simulink model "sim_UAV_Cascada"  (R2015a)
settings: Solver=ode45  StartTime=0.0  StopTime=20  MaxStep=0.001  RelTol=1e-3
values from neighbouring files (symbols this model uses):
  g = 9.81    [Init_UAV.m]    (also in Parametros.m)
  K_pitch = 0.1861    [Parametros.m]
  K_roll = 0.1861    [Parametros.m]
  K_yaw = 2.48    [Parametros.m]
  Kd_pitch = 0.0957    [Parametros.m]
  Kd_roll = 0.0957    [Parametros.m]
  Kd_yaw = 0    [Parametros.m]
  Ki_pitch = 3.69    [Parametros.m]
  Ki_roll = 3.69    [Parametros.m]
  Ki_yaw = 3.77    [Parametros.m]
  KKt = 0.8    [Parametros.m]
  Kphi = 0.4    [Parametros.m]
  Kpsi = 0.3    [Parametros.m]
  Ktheta = 0.4    [Parametros.m]
  l = 0.235    [Init_UAV.m]    (also in Parametros.m)
  m = 0.65    [Init_UAV.m]    (also in Parametros.m = 1.3)
  N = 18    [Parametros.m]
  Nyaw = 10    [Parametros.m]
  tau = 0.06035    [Parametros.m]
  Tt = 1    [Parametros.m]
  Ttyaw = 3.5    [Parametros.m]
undefined symbols (not defined in the file): attitude0, I, omega0, pos0, vel0
libraries: simulink x12, aerolibtransform2 x2, aerolibutil x2
settings Model: Creator=Miguel  LastModifiedBy=Eduardo
settings DataIOCC: SignalLoggingSaveFormat=ModelDataLogs
settings DebuggingCC: SolverPrmCheckMsg=warning  MultiTaskDSMMsg=warning  MultiTaskCondExecSysMsg=none  StrictBusMsg=ErrorOnBusTreatedAsVector

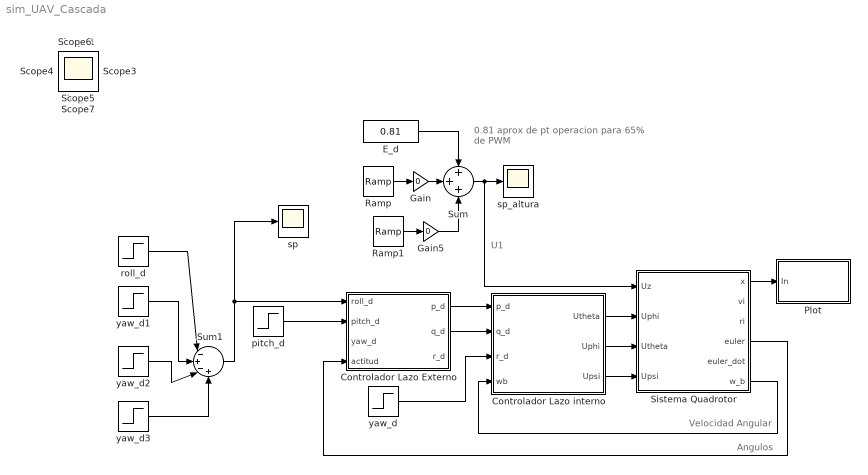
== system sim_UAV_Cascada ==
  note: U1
  note: Angulos
  note: Velocidad Angular
  note: 0.81 aprox
      | de pt operacion para 65% de PWM
  Controlador Lazo Externo : Subsystem
  "Controlador Lazo interno " : Subsystem
  E_d : Constant  Value=0.81
  Gain : Gain  Gain=0
  Gain5 : Gain  Gain=0
  Plot : Subsystem
  Ramp : simulink/Sources/Ramp  slope=1  start=3  X0=0
  Ramp1 : simulink/Sources/Ramp  slope=-1  start=13  X0=0
  Sistema Quadrotor : Subsystem
  Sum : Sum  Inputs=+++
  Sum1 : Sum  Inputs=|-+-+
  pitch_d : Step  Time=0  After=0  SampleTime=0
  roll_d : Step  Time=5  After=25  SampleTime=0
  sp : Scope
      settings: TimeRange=3.666361136571954  YMin=-12.33117816091954  YMax=-8.609913793103445  SaveName=ScopeData21
  sp_altura : Scope
      settings: TimeRange=3.666361136571954  YMin=-12.33117816091954  YMax=-8.609913793103445  SaveName=ScopeData19
  yaw_d : Step  Time=3  After=0  SampleTime=0
  yaw_d1 : Step  Time=7  After=55  SampleTime=0
  yaw_d2 : Step  Time=12  After=50  SampleTime=0
  yaw_d3 : Step  Time=16  After=20  SampleTime=0
  Scope{,1..7} (8 alike) : Scope
      Scope settings: MaxDataPoints=7500
      Scope1 settings: MaxDataPoints=7500
      Scope2 settings: SaveName=ScopeData2  MaxDataPoints=7500
      Scope3 settings: SaveName=ScopeData3  MaxDataPoints=7500
      Scope4 settings: SaveName=ScopeData4  MaxDataPoints=7500
      Scope5 settings: SaveName=ScopeData5  MaxDataPoints=7500
      Scope6 settings: SaveName=ScopeData6  MaxDataPoints=7500
      Scope7 settings: SaveName=ScopeData7  MaxDataPoints=7500
  wires:
  Sistema Quadrotor/1(x) -> Plot/1(In)
  Controlador Lazo Externo/1(p_d) -> "Controlador Lazo interno "/1(p_d)
  Controlador Lazo Externo/2(q_d) -> "Controlador Lazo interno "/2(q_d)
  pitch_d/1 -> Controlador Lazo Externo/2(pitch_d)
  yaw_d1/1 -> Sum1/2
  yaw_d2/1 -> Sum1/3
  yaw_d3/1 -> Sum1/4
  Sistema Quadrotor/6(w_b) -> "Controlador Lazo interno "/4(wb)
  Sistema Quadrotor/4(euler) -> Controlador Lazo Externo/4(actitud)
  E_d/1 -> Sum/1
  Sum/1 -> Sistema Quadrotor/1(Uz), sp_altura/1
  Gain/1 -> Sum/2
  Ramp/1 -> Gain/1
  Ramp1/1 -> Gain5/1
  Gain5/1 -> Sum/3
  "Controlador Lazo interno "/1(Utheta) -> Sistema Quadrotor/2(Uphi)
  "Controlador Lazo interno "/2(Uphi) -> Sistema Quadrotor/3("Utheta ")
  "Controlador Lazo interno "/3(Upsi) -> Sistema Quadrotor/4(Upsi)
  Sum1/1 -> Controlador Lazo Externo/1(roll_d), sp/1
  yaw_d/1 -> "Controlador Lazo interno "/3(r_d)
  roll_d/1 -> Sum1/1

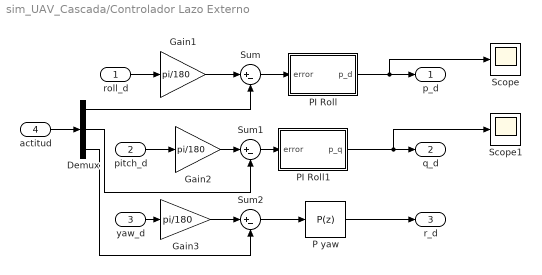
== system sim_UAV_Cascada/Controlador Lazo Externo ==
  roll_d : Inport
  pitch_d : Inport  Port=2
  yaw_d : Inport  Port=3
  actitud : Inport  Port=4
  Demux : Demux  Outputs=3
  Gain1 : Gain  Gain=pi/180
  Gain2 : Gain  Gain=pi/180
  Gain3 : Gain  Gain=pi/180
  P yaw : simulink/Continuous/PID Controller  Controller=P  TimeDomain=Discrete-time  SampleTime=0.01  IntegratorMethod=Forward Euler  FilterMethod=Forward Euler  Form=Parallel  UseFilter=on  ControllerParametersSource=internal  P=4  I=1.5  D=0.00989768140502374  N=2166.61961334261  InitialConditionSource=internal  InitialConditionForIntegrator=0  InitialConditionForFilter=0  ExternalReset=none  LimitOutput=off  UpperSaturationLimit=1.555  LowerSaturationLimit=-1.552  LinearizeAsGain=on  AntiWindupMode=back-calculation  Kb=1  TrackingMode=off  Kt=1  PParamMin=[]  PParamMax=[]  IParamMin=[]  IParamMax=[]  DParamMin=[]  DParamMax=[]  NParamMin=[]  NParamMax=[]  KbParamMin=[]  KbParamMax=[]  KtParamMin=[]  KtParamMax=[]  POutMin=[]  POutMax=[]  IOutMin=[]  IOutMax=[]  DOutMin=[]  DOutMax=[]  NOutMin=[]  NOutMax=[]  KbOutMin=[]  KbOutMax=[]  KtOutMin=[]  KtOutMax=[]  IntegratorOutMin=[]  IntegratorOutMax=[]  FilterOutMin=[]  FilterOutMax=[]  SumOutMin=[]  SumOutMax=[]  SumI1OutMin=[]  SumI1OutMax=[]  SumI2OutMin=[]  SumI2OutMax=[]  SumI3OutMin=[]  SumI3OutMax=[]  SumDOutMin=[]  SumDOutMax=[]  SaturationOutMin=[]  SaturationOutMax=[]  IntegratorContinuousStateAttributes=''  IntegratorStateMustResolveToSignalObject=off  IntegratorRTWStateStorageClass=Auto  FilterContinuousStateAttributes=''  FilterStateMustResolveToSignalObject=off  FilterRTWStateStorageClass=Auto  DifferentiatorICPrevScaledInput=0  DifferentiatorOutMin=[]  DifferentiatorOutMax=[]
  PI Roll : Subsystem
  PI Roll1 : Subsystem
  Scope : Scope
      settings: SaveName=ScopeData27
  Scope1 : Scope
      settings: SaveName=ScopeData28
  Sum : Sum  Inputs=|+-
  Sum1 : Sum  Inputs=|+-
  Sum2 : Sum  Inputs=|+-
  p_d : Outport
  q_d : Outport  Port=2
  r_d : Outport  Port=3
  wires:
  PI Roll1/1(p_q) -> Scope1/1, q_d/1
  P yaw/1 -> r_d/1
  actitud/1 -> Demux/1
  roll_d/1 -> Gain1/1
  pitch_d/1 -> Gain2/1
  yaw_d/1 -> Gain3/1
  Demux/1 -> Sum/2
  Demux/2 -> Sum1/2
  Demux/3 -> Sum2/2
  Sum2/1 -> P yaw/1
  Gain1/1 -> Sum/1
  Gain2/1 -> Sum1/1
  Gain3/1 -> Sum2/1
  Sum/1 -> PI Roll/1(error)
  PI Roll/1(p_d) -> Scope/1, p_d/1
  Sum1/1 -> PI Roll1/1(error)

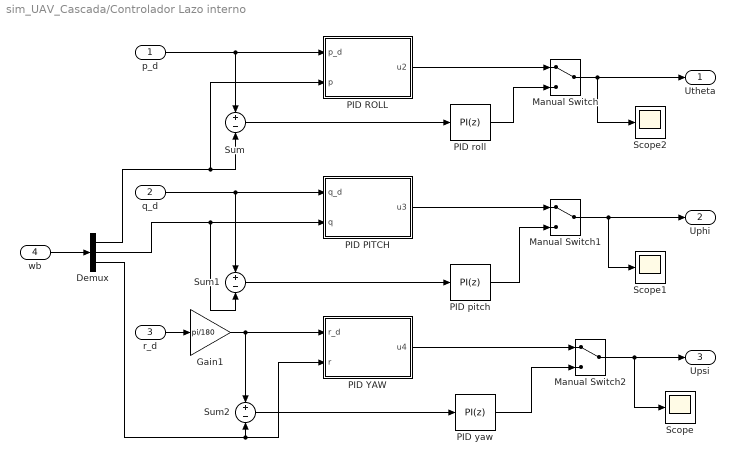
== system sim_UAV_Cascada/Controlador Lazo interno  ==
  p_d : Inport
  q_d : Inport  Port=2
  r_d : Inport  Port=3
  wb : Inport  Port=4
  Demux : Demux  Outputs=3
  Gain1 : Gain  Gain=pi/180
  Manual Switch : ManualSwitch
  Manual Switch1 : ManualSwitch
  Manual Switch2 : ManualSwitch
  PID PITCH : Subsystem
  PID ROLL : Subsystem
  PID YAW : Subsystem
  PID pitch : simulink/Continuous/PID Controller  Controller=PI  TimeDomain=Discrete-time  SampleTime=0.01  IntegratorMethod=Forward Euler  FilterMethod=Forward Euler  Form=Ideal  UseFilter=on  ControllerParametersSource=internal  P=0.09  I=1/0.85  D=0.08  N=10  InitialConditionSource=internal  InitialConditionForIntegrator=0  InitialConditionForFilter=0  ExternalReset=none  LimitOutput=on  UpperSaturationLimit=1  LowerSaturationLimit=-1  LinearizeAsGain=on  AntiWindupMode=back-calculation  Kb=1  TrackingMode=off  Kt=1  PParamMin=[]  PParamMax=[]  IParamMin=[]  IParamMax=[]  DParamMin=[]  DParamMax=[]  NParamMin=[]  NParamMax=[]  KbParamMin=[]  KbParamMax=[]  KtParamMin=[]  KtParamMax=[]  POutMin=[]  POutMax=[]  IOutMin=[]  IOutMax=[]  DOutMin=[]  DOutMax=[]  NOutMin=[]  NOutMax=[]  KbOutMin=[]  KbOutMax=[]  KtOutMin=[]  KtOutMax=[]  IntegratorOutMin=[]  IntegratorOutMax=[]  FilterOutMin=[]  FilterOutMax=[]  SumOutMin=[]  SumOutMax=[]  SumI1OutMin=[]  SumI1OutMax=[]  SumI2OutMin=[]  SumI2OutMax=[]  SumI3OutMin=[]  SumI3OutMax=[]  SumDOutMin=[]  SumDOutMax=[]  SaturationOutMin=[]  SaturationOutMax=[]  IntegratorContinuousStateAttributes=''  IntegratorStateMustResolveToSignalObject=off  IntegratorRTWStateStorageClass=Auto  FilterContinuousStateAttributes=''  FilterStateMustResolveToSignalObject=off  FilterRTWStateStorageClass=Auto  DifferentiatorICPrevScaledInput=0  DifferentiatorOutMin=[]  DifferentiatorOutMax=[]
  PID roll : simulink/Continuous/PID Controller  Controller=PI  TimeDomain=Discrete-time  SampleTime=0.01  IntegratorMethod=Forward Euler  FilterMethod=Forward Euler  Form=Ideal  UseFilter=on  ControllerParametersSource=internal  P=0.09  I=1/0.85  D=0.025  N=10  InitialConditionSource=internal  InitialConditionForIntegrator=0  InitialConditionForFilter=0  ExternalReset=none  LimitOutput=on  UpperSaturationLimit=1  LowerSaturationLimit=-1  LinearizeAsGain=on  AntiWindupMode=back-calculation  Kb=1  TrackingMode=off  Kt=1  PParamMin=[]  PParamMax=[]  IParamMin=[]  IParamMax=[]  DParamMin=[]  DParamMax=[]  NParamMin=[]  NParamMax=[]  KbParamMin=[]  KbParamMax=[]  KtParamMin=[]  KtParamMax=[]  POutMin=[]  POutMax=[]  IOutMin=[]  IOutMax=[]  DOutMin=[]  DOutMax=[]  NOutMin=[]  NOutMax=[]  KbOutMin=[]  KbOutMax=[]  KtOutMin=[]  KtOutMax=[]  IntegratorOutMin=[]  IntegratorOutMax=[]  FilterOutMin=[]  FilterOutMax=[]  SumOutMin=[]  SumOutMax=[]  SumI1OutMin=[]  SumI1OutMax=[]  SumI2OutMin=[]  SumI2OutMax=[]  SumI3OutMin=[]  SumI3OutMax=[]  SumDOutMin=[]  SumDOutMax=[]  SaturationOutMin=[]  SaturationOutMax=[]  IntegratorContinuousStateAttributes=''  IntegratorStateMustResolveToSignalObject=off  IntegratorRTWStateStorageClass=Auto  FilterContinuousStateAttributes=''  FilterStateMustResolveToSignalObject=off  FilterRTWStateStorageClass=Auto  DifferentiatorICPrevScaledInput=0  DifferentiatorOutMin=[]  DifferentiatorOutMax=[]
  PID yaw : simulink/Continuous/PID Controller  Controller=PI  TimeDomain=Discrete-time  SampleTime=0.01  IntegratorMethod=Forward Euler  FilterMethod=Forward Euler  Form=Ideal  UseFilter=on  ControllerParametersSource=internal  P=2.48  I=0.26  D=0.09571  N=189.5  InitialConditionSource=internal  InitialConditionForIntegrator=0  InitialConditionForFilter=0  ExternalReset=none  LimitOutput=on  UpperSaturationLimit=1  LowerSaturationLimit=-1  LinearizeAsGain=on  AntiWindupMode=back-calculation  Kb=3.5  TrackingMode=off  Kt=1  PParamMin=[]  PParamMax=[]  IParamMin=[]  IParamMax=[]  DParamMin=[]  DParamMax=[]  NParamMin=[]  NParamMax=[]  KbParamMin=[]  KbParamMax=[]  KtParamMin=[]  KtParamMax=[]  POutMin=[]  POutMax=[]  IOutMin=[]  IOutMax=[]  DOutMin=[]  DOutMax=[]  NOutMin=[]  NOutMax=[]  KbOutMin=[]  KbOutMax=[]  KtOutMin=[]  KtOutMax=[]  IntegratorOutMin=[]  IntegratorOutMax=[]  FilterOutMin=[]  FilterOutMax=[]  SumOutMin=[]  SumOutMax=[]  SumI1OutMin=[]  SumI1OutMax=[]  SumI2OutMin=[]  SumI2OutMax=[]  SumI3OutMin=[]  SumI3OutMax=[]  SumDOutMin=[]  SumDOutMax=[]  SaturationOutMin=[]  SaturationOutMax=[]  IntegratorContinuousStateAttributes=''  IntegratorStateMustResolveToSignalObject=off  IntegratorRTWStateStorageClass=Auto  FilterContinuousStateAttributes=''  FilterStateMustResolveToSignalObject=off  FilterRTWStateStorageClass=Auto  DifferentiatorICPrevScaledInput=0  DifferentiatorOutMin=[]  DifferentiatorOutMax=[]
  Scope : Scope
      settings: YMin=0.13  YMax=0.36  SaveName=ScopeData13
  Scope1 : Scope
      settings: SaveName=ScopeData14
  Scope2 : Scope
      settings: TimeRange=16  YMin=0  YMax=0.00014  SaveName=ScopeData15
  Sum : Sum  Inputs=+-
  Sum1 : Sum  Inputs=+-
  Sum2 : Sum  Inputs=+-
  Utheta : Outport
  Uphi : Outport  Port=2
  Upsi : Outport  Port=3
  wires:
  Manual Switch2/1 -> Upsi/1, Scope/1
  Manual Switch/1 -> Utheta/1, Scope2/1
  Manual Switch1/1 -> Uphi/1, Scope1/1
  wb/1 -> Demux/1
  p_d/1 -> PID ROLL/1(p_d), Sum/1
  q_d/1 -> Sum1/1, PID PITCH/1(q_d)
  Demux/1 -> PID ROLL/2(p), Sum/2
  Demux/2 -> Sum1/2, PID PITCH/2(q)
  Demux/3 -> PID YAW/2(r), Sum2/2
  Sum/1 -> PID roll/1
  PID pitch/1 -> Manual Switch1/2
  Sum1/1 -> PID pitch/1
  Sum2/1 -> PID yaw/1
  PID yaw/1 -> Manual Switch2/2
  PID roll/1 -> Manual Switch/2
  PID PITCH/1(u3) -> Manual Switch1/1
  PID ROLL/1(u2) -> Manual Switch/1
  PID YAW/1(u4) -> Manual Switch2/1
  r_d/1 -> Gain1/1
  Gain1/1 -> Sum2/1, PID YAW/1(r_d)

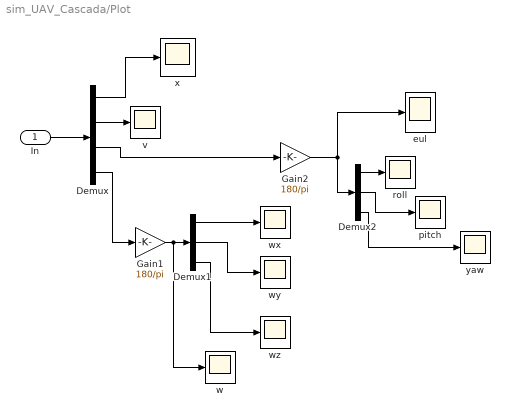
== system sim_UAV_Cascada/Plot ==
  In : Inport
  Demux : Demux
  Demux1 : Demux  Outputs=3
  Demux2 : Demux  Outputs=3
  Gain1 : Gain  Gain=180/pi
  Gain2 : Gain  Gain=180/pi
  eul : Scope
      settings: TimeRange=8  SaveName=ScopeData2
  pitch : Scope
      settings: TimeRange=10  YMin=-0.01  YMax=0.09000000000000001  SaveName=ScopeData12
  roll : Scope
      settings: SaveName=ScopeData10
  v : Scope
  w : Scope
      settings: SaveName=ScopeData25
  wx : Scope
      settings: SaveName=ScopeData3
  wy : Scope
      settings: SaveName=ScopeData23
  wz : Scope
      settings: SaveName=ScopeData24
  x : Scope
  yaw : Scope
      settings: SaveName=ScopeData11
  wires:
  In/1 -> Demux/1
  Demux/1 -> x/1
  Demux/2 -> v/1
  Demux/3 -> Gain2/1
  Gain2/1 -> eul/1, Demux2/1
  Demux2/1 -> roll/1
  Demux2/2 -> pitch/1
  Demux2/3 -> yaw/1
  Demux/4 -> Gain1/1
  Demux1/1 -> wx/1
  Gain1/1 -> w/1, Demux1/1
  Demux1/2 -> wy/1
  Demux1/3 -> wz/1

== system sim_UAV_Cascada/Sistema Quadrotor ==
  Uz : Inport
  Uphi : Inport  Port=2
  "Utheta " : Inport  Port=3
  Upsi : Inport  Port=4
  ACTUADORES : Subsystem
  AERODINÁMICAS : Subsystem
  DINÁMICA QUADROTOR : Subsystem
      mask Display:
      | image(imread('F450.jpg'))
      | port_label('input',1,'{F}^{b} (N)','texmode','on')
      | port_label('input',2,'{M}^{b} (N-m)','texmode','on')
      | port_label('output',1,'x ','texmode','on')
      | port_label('output',2,'{v}^{i} (m/s)','texmode','on')
      | port_label('output',3,'{r}^{i} (m)','texmode','on')
      | port_label('output',4,'\phi \theta \psi (rad)','texmode','on')
      | port_label('output',5,'d[\phi \theta \psi]/dt (rad)','texmode','on')
  MATRIZ DE CONVERSION PWM : Subsystem
  x : Outport
  vi : Outport  Port=2
  ri : Outport  Port=3
  euler : Outport  Port=4
  euler_dot : Outport  Port=5
  w_b : Outport  Port=6
  wires:
  DINÁMICA QUADROTOR/2(v) -> vi/1
  DINÁMICA QUADROTOR/1(estados) -> x/1
  DINÁMICA QUADROTOR/4(eul) -> euler/1
  ACTUADORES/1(Ti) -> AERODINÁMICAS/1(Ti)
  AERODINÁMICAS/1(Fb) -> DINÁMICA QUADROTOR/1(Fuerza)
  AERODINÁMICAS/2(Mb) -> DINÁMICA QUADROTOR/2(Momento)
  DINÁMICA QUADROTOR/3(pos) -> ri/1
  DINÁMICA QUADROTOR/5(Deul) -> euler_dot/1
  DINÁMICA QUADROTOR/6(w_b) -> w_b/1
  ACTUADORES/2(Mi) -> AERODINÁMICAS/2(Mi)
  Uphi/1 -> MATRIZ DE CONVERSION PWM/2(Uphi)
  Uz/1 -> MATRIZ DE CONVERSION PWM/1(Uz)
  "Utheta "/1 -> MATRIZ DE CONVERSION PWM/3(Utheta)
  Upsi/1 -> MATRIZ DE CONVERSION PWM/4(Upsi)
  MATRIZ DE CONVERSION PWM/1(PWM%) -> ACTUADORES/1(PWM%)

== system sim_UAV_Cascada/Controlador Lazo Externo/PI Roll ==
  note: error
  error : Inport
  Integrator : Integrator
  K : Gain  Gain=6
  Sum6 : Sum  Inputs=|++
  Ti : Gain  Gain=0.5
  p_d : Outport
  wires:
  error/1 -> Ti/1, K/1
  K/1 -> Sum6/1
  Ti/1 -> Integrator/1
  Integrator/1 -> Sum6/2
  Sum6/1 -> p_d/1

== system sim_UAV_Cascada/Controlador Lazo Externo/PI Roll1 ==
  note: error
  error : Inport
  Integrator : Integrator
  K : Gain  Gain=6
  Sum6 : Sum  Inputs=|++
  Ti : Gain  Gain=0.5
  p_q : Outport
  wires:
  error/1 -> Ti/1, K/1
  K/1 -> Sum6/1
  Ti/1 -> Integrator/1
  Integrator/1 -> Sum6/2
  Sum6/1 -> p_q/1

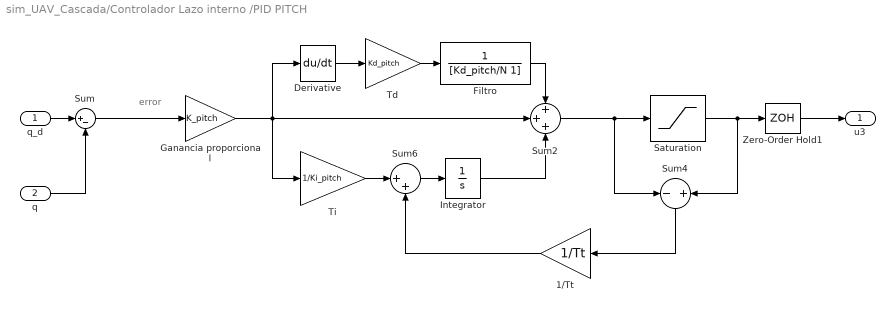
== system sim_UAV_Cascada/Controlador Lazo interno /PID PITCH ==
  note: error
  q_d : Inport
  q : Inport  Port=2
  1/Tt : Gain  Gain=1/Tt
  Derivative : Derivative
  Filtro : TransferFcn  Denominator=[Kd_pitch/N 1]
  Ganancia proporcional : Gain  Gain=K_pitch
  Integrator : Integrator
  Saturation : Saturate  UpperLimit=1  LowerLimit=-1
  Sum : Sum  Inputs=|+-
  Sum2 : Sum  Inputs=+++
  Sum4 : Sum  Inputs=-|+
  Sum6 : Sum  Inputs=|++
  Td : Gain  Gain=Kd_pitch
  Ti : Gain  Gain=1/Ki_pitch
  Zero-Order Hold1 : ZeroOrderHold  SampleTime=0.01
  u3 : Outport
  wires:
  q/1 -> Sum/2
  Sum6/1 -> Integrator/1
  Ganancia proporcional/1 -> Sum2/2, Derivative/1, Ti/1
  Derivative/1 -> Td/1
  Sum4/1 -> 1/Tt/1
  Saturation/1 -> Sum4/2, Zero-Order Hold1/1
  Sum2/1 -> Sum4/1, Saturation/1
  q_d/1 -> Sum/1
  Sum/1 -> Ganancia proporcional/1
  Ti/1 -> Sum6/1
  1/Tt/1 -> Sum6/2
  Td/1 -> Filtro/1
  Integrator/1 -> Sum2/3
  Filtro/1 -> Sum2/1
  Zero-Order Hold1/1 -> u3/1

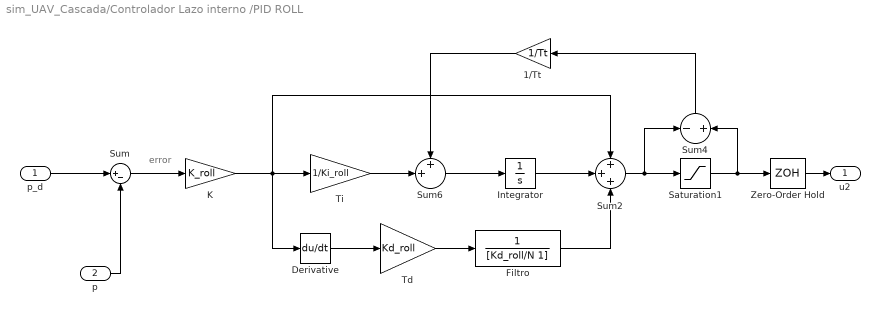
== system sim_UAV_Cascada/Controlador Lazo interno /PID ROLL ==
  note: error
  p_d : Inport
  p : Inport  Port=2
  1/Tt : Gain  Gain=1/Tt
  Derivative : Derivative
  Filtro : TransferFcn  Denominator=[Kd_roll/N 1]
  Integrator : Integrator
  K : Gain  Gain=K_roll
  Saturation1 : Saturate  UpperLimit=1  LowerLimit=-1
  Sum : Sum  Inputs=|+-
  Sum2 : Sum  Inputs=+++
  Sum4 : Sum  Inputs=-+
  Sum6 : Sum  Inputs=++|
  Td : Gain  Gain=Kd_roll
  Ti : Gain  Gain=1/Ki_roll
  Zero-Order Hold : ZeroOrderHold  SampleTime=0.01
  u2 : Outport
  wires:
  p/1 -> Sum/2
  1/Tt/1 -> Sum6/1
  Sum6/1 -> Integrator/1
  K/1 -> Derivative/1, Ti/1, Sum2/1
  Derivative/1 -> Td/1
  Filtro/1 -> Sum2/3
  Td/1 -> Filtro/1
  Integrator/1 -> Sum2/2
  Ti/1 -> Sum6/2
  Sum4/1 -> 1/Tt/1
  Sum2/1 -> Sum4/1, Saturation1/1
  p_d/1 -> Sum/1
  Sum/1 -> K/1
  Saturation1/1 -> Sum4/2, Zero-Order Hold/1
  Zero-Order Hold/1 -> u2/1

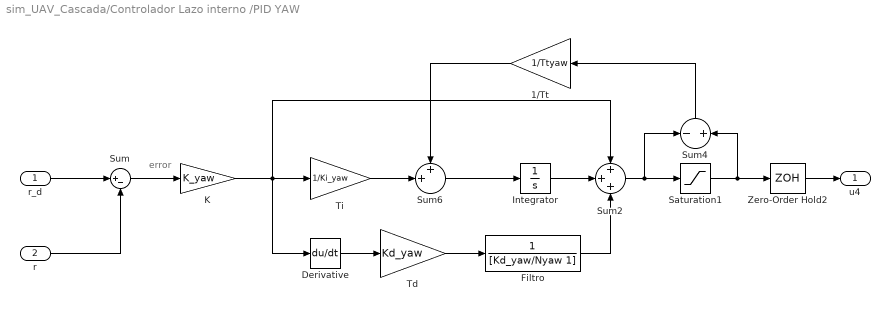
== system sim_UAV_Cascada/Controlador Lazo interno /PID YAW ==
  note: error
  r_d : Inport
  r : Inport  Port=2
  1/Tt : Gain  Gain=1/Ttyaw
  Derivative : Derivative
  Filtro : TransferFcn  Denominator=[Kd_yaw/Nyaw 1]
  Integrator : Integrator
  K : Gain  Gain=K_yaw
  Saturation1 : Saturate  UpperLimit=1  LowerLimit=-1
  Sum : Sum  Inputs=|+-
  Sum2 : Sum  Inputs=+++
  Sum4 : Sum  Inputs=-+
  Sum6 : Sum  Inputs=++|
  Td : Gain  Gain=Kd_yaw
  Ti : Gain  Gain=1/Ki_yaw
  Zero-Order Hold2 : ZeroOrderHold  SampleTime=0.01
  u4 : Outport
  wires:
  r/1 -> Sum/2
  1/Tt/1 -> Sum6/1
  Sum6/1 -> Integrator/1
  K/1 -> Derivative/1, Ti/1, Sum2/1
  Derivative/1 -> Td/1
  Filtro/1 -> Sum2/3
  Td/1 -> Filtro/1
  Integrator/1 -> Sum2/2
  Ti/1 -> Sum6/2
  Sum4/1 -> 1/Tt/1
  Saturation1/1 -> Zero-Order Hold2/1, Sum4/2
  Sum2/1 -> Sum4/1, Saturation1/1
  r_d/1 -> Sum/1
  Sum/1 -> K/1
  Zero-Order Hold2/1 -> u4/1

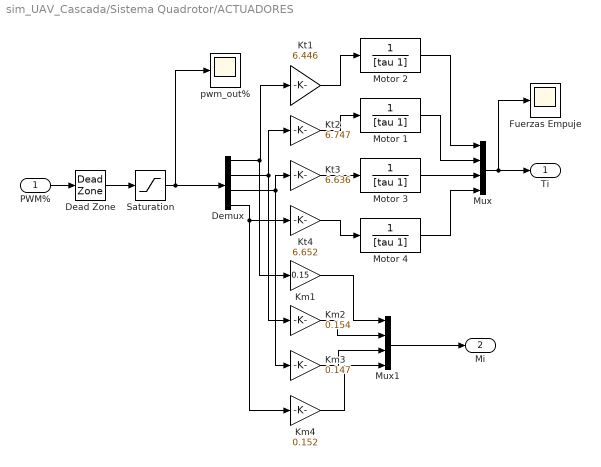
== system sim_UAV_Cascada/Sistema Quadrotor/ACTUADORES ==
  PWM% : Inport
  Dead Zone : DeadZone  LowerValue=0  UpperValue=0.13  SaturateOnIntegerOverflow=on
  Demux : Demux
  Fuerzas Empuje : Scope
      settings: SaveName=ScopeData20
  Km1 : Gain  Gain=0.15
  Km2 : Gain  Gain=0.154
  Km3 : Gain  Gain=0.147
  Km4 : Gain  Gain=0.152
  Kt1 : Gain  Gain=6.446
  Kt2 : Gain  Gain=6.747
  Kt3 : Gain  Gain=6.636
  Kt4 : Gain  Gain=6.652
  Motor {1..4} (4 alike) : TransferFcn  Denominator=[tau 1]
  Mux : Mux
  Mux1 : Mux
  Saturation : Saturate  UpperLimit=1  LowerLimit=0  ZeroCross=off
  pwm_out% : Scope
      settings: SaveName=ScopeData22
  Ti : Outport
  Mi : Outport  Port=2
  wires:
  PWM%/1 -> Dead Zone/1
  Dead Zone/1 -> Saturation/1
  Saturation/1 -> Demux/1, pwm_out%/1
  Demux/1 -> Km1/1, Kt1/1
  Demux/2 -> Km2/1, Kt2/1
  Demux/3 -> Kt3/1, Km3/1
  Demux/4 -> Km4/1, Kt4/1
  Km1/1 -> Mux1/1
  Km2/1 -> Mux1/2
  Km3/1 -> Mux1/3
  Km4/1 -> Mux1/4
  Mux1/1 -> Mi/1
  Kt4/1 -> Motor 4/1
  Kt3/1 -> Motor 3/1
  Kt2/1 -> Motor 1/1
  Kt1/1 -> Motor 2/1
  Motor 2/1 -> Mux/1
  Motor 1/1 -> Mux/2
  Motor 3/1 -> Mux/3
  Motor 4/1 -> Mux/4
  Mux/1 -> Fuerzas Empuje/1, Ti/1

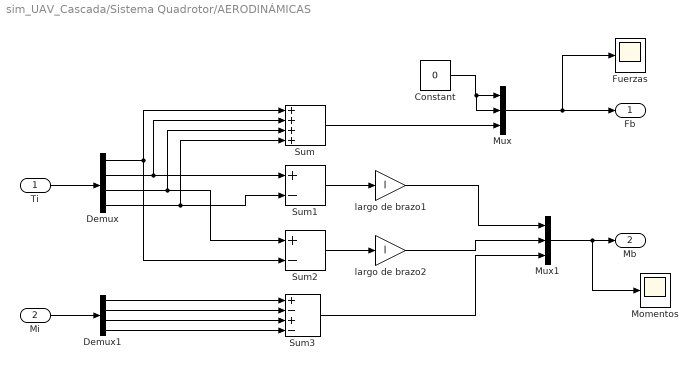
== system sim_UAV_Cascada/Sistema Quadrotor/AERODINÁMICAS ==
  Ti : Inport
  Mi : Inport  Port=2
  Constant : Constant  Value=0
  Demux : Demux
  Demux1 : Demux
  Fuerzas : Scope
      settings: SaveName=ScopeData4
  Momentos : Scope
      settings: SaveName=ScopeData8
  Mux : Mux  Inputs=3
  Mux1 : Mux  Inputs=3
  Sum : Sum  Inputs=++++
  Sum1 : Sum  Inputs=+-
  Sum2 : Sum  Inputs=+-
  Sum3 : Sum  Inputs=+-+-
  largo de brazo1 : Gain  Gain=l
  largo de brazo2 : Gain  Gain=l
  Fb : Outport
  Mb : Outport  Port=2
  wires:
  Ti/1 -> Demux/1
  Mi/1 -> Demux1/1
  Demux/1 -> Sum2/2, Sum/1
  Demux/2 -> Sum1/1, Sum/2
  Demux/3 -> Sum2/1, Sum/3
  Demux/4 -> Sum1/2, Sum/4
  Demux1/1 -> Sum3/1
  Demux1/2 -> Sum3/2
  Demux1/3 -> Sum3/3
  Demux1/4 -> Sum3/4
  Sum1/1 -> largo de brazo1/1
  Sum2/1 -> largo de brazo2/1
  Constant/1 -> Mux/2, Mux/1
  Mux/1 -> Fb/1, Fuerzas/1
  Sum/1 -> Mux/3
  largo de brazo1/1 -> Mux1/1
  largo de brazo2/1 -> Mux1/2
  Sum3/1 -> Mux1/3
  Mux1/1 -> Momentos/1, Mb/1

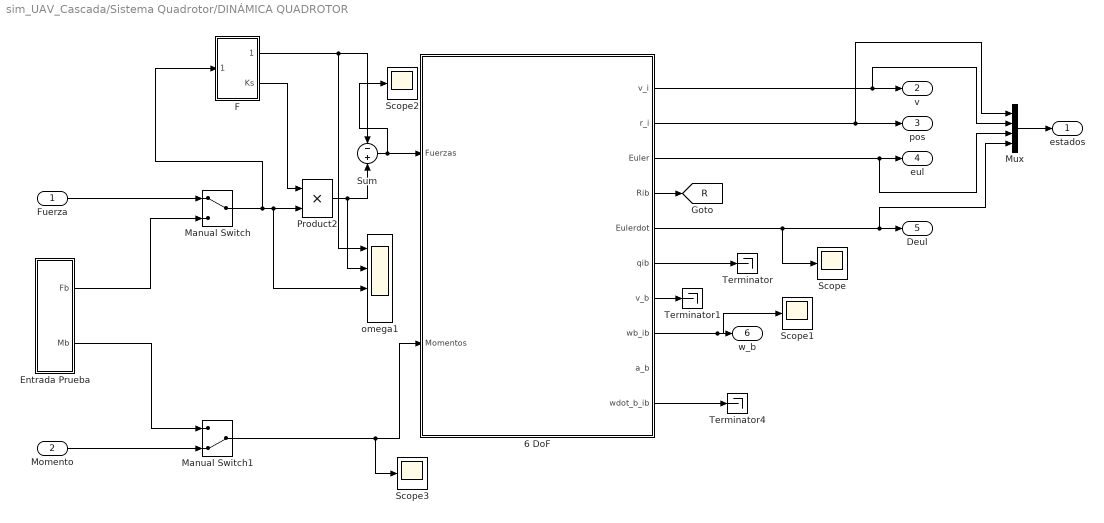
== system sim_UAV_Cascada/Sistema Quadrotor/DINÁMICA QUADROTOR ==
  Fuerza : Inport
  Momento : Inport  Port=2
  6 DoF : Subsystem  mask(Sistema Cuadrirotor){masa=m, Inercia=I, v0_b=vel0, w0b_ib=omega0, r0_i=pos0, eul_0=attitude0}
      mask prompts: masa "masa (Kg) :"; Inercia "Inercia :"; v0_b "Velocidad lineal inicial en el body (m/s):"; w0b_ib "Velocidad angular inicial en el body (rad/s) :"; r0_i "Posición inicial en el inercial (m) :"; eul_0 "Angulos de euler iniciales"
      mask help: Modelo cinemático y dinámico de un UAV tipo Cuadrirotor
      mask Display:
      | port_label('input',1,'{F}^{b} (N)','texmode','on')
      | port_label('input',2,'{M}^{b} (N-m)','texmode','on')
      | port_label('output',1,'{v}^{i} (m/s)','texmode','on')
      | port_label('output',2,'{r}^{i} (m)','texmode','on')
      | port_label('output',3,'\phi \theta \psi (rad)','texmode','on')
      | port_label('output',4,'{R}^{i}_{b}','texmode','on')
      | port_label('output',5,'d[\phi \theta \psi]/dt (rad)','texmode','on')
      | port_label('output',6,'{q}^{i}_{b}','texmode','on')
      | port_label('output',7,'{v}^{b} (m/s)','texmode','on')
      | port_label('output',8,'{\omega}^{b}_{bi} (rad)','texmode','on')
      | port_label('output',9,'{a}^{b} (m/{s}^{2})','texmode','on')
      | port_label('output',10,'d({\omega}^{b}_{ib})/dt (rad/{s}^{2})','texmode','on')
  Entrada Prueba : Subsystem
  F : Subsystem
  Manual Switch : ManualSwitch
  Manual Switch1 : ManualSwitch  CurrentSetting=0
  Mux : Mux
  Product2 : Product
  Scope{,1..3} (4 alike) : Scope
      Scope settings: SaveName=ScopeData16
      Scope1 settings: SaveName=ScopeData17
      Scope2 settings: SaveName=ScopeData18
      Scope3 settings: SaveName=ScopeData26
  Sum : Sum  Inputs=-|+
  Terminator : Terminator
  Terminator1 : Terminator
  Terminator4 : Terminator
  omega1 : Scope  NumInputPorts=4
      settings: YMin=-1~-20~-20~-5  YMax=12~0~0~5  SaveName=ScopeData9
  estados : Outport
  v : Outport  Port=2
  pos : Outport  Port=3
  eul : Outport  Port=4
  Deul : Outport  Port=5
  w_b : Outport  Port=6
  tag scope: R=global
  wires:
  6 DoF/2(r_i) -> pos/1, Mux/1
  6 DoF/4(Rib) -> [R]
  6 DoF/6(qib) -> Terminator/1
  6 DoF/5(Eulerdot) -> Mux/4, Deul/1, Scope/1
  6 DoF/3(Euler) -> Mux/3, eul/1
  Sum/1 -> Scope2/1, 6 DoF/1(Fuerzas)
  6 DoF/10(wdot_b_ib) -> Terminator4/1
  6 DoF/1(v_i) -> Mux/2, v/1
  6 DoF/7(v_b) -> Terminator1/1
  6 DoF/8(wb_ib) -> Scope1/1, w_b/1
  Mux/1 -> estados/1
  Entrada Prueba/1(Fb) -> Manual Switch/2
  Entrada Prueba/2(Mb) -> Manual Switch1/1
  Fuerza/1 -> Manual Switch/1
  Momento/1 -> Manual Switch1/2
  Manual Switch1/1 -> Scope3/1, 6 DoF/2(Momentos)
  Manual Switch/1 -> omega1/3, Product2/2, F/1(Fm_b)
  F/1(Fg_b) -> omega1/1, Sum/1
  Product2/1 -> omega1/2, Sum/2
  F/2(Ks) -> Product2/1

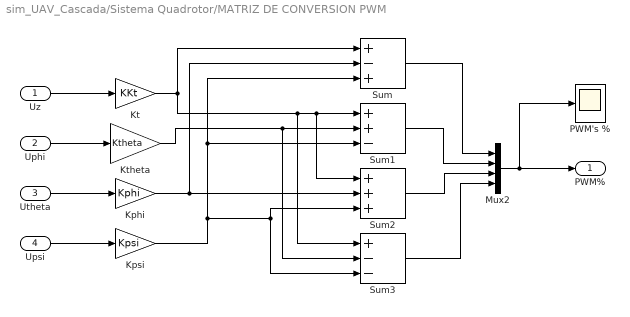
== system sim_UAV_Cascada/Sistema Quadrotor/MATRIZ DE CONVERSION PWM ==
  Uz : Inport
  Uphi : Inport  Port=2
  Utheta : Inport  Port=3
  Upsi : Inport  Port=4
  Kphi : Gain  Gain=Kphi
  Kpsi : Gain  Gain=Kpsi
  Kt : Gain  Gain=KKt
  Ktheta : Gain  Gain=Ktheta
  Mux2 : Mux
  PWM's % : Scope
  Sum : Sum  Inputs=+-+
  Sum1 : Sum  Inputs=++-
  Sum2 : Sum  Inputs=+++
  Sum3 : Sum  Inputs=+--
  PWM% : Outport
  wires:
  Sum/1 -> Mux2/1
  Sum1/1 -> Mux2/2
  Sum2/1 -> Mux2/3
  Sum3/1 -> Mux2/4
  Uz/1 -> Kt/1
  Mux2/1 -> PWM%/1, PWM's %/1
  Uphi/1 -> Ktheta/1
  Utheta/1 -> Kphi/1
  Upsi/1 -> Kpsi/1
  Kt/1 -> Sum1/1, Sum2/1, Sum3/1, Sum/1
  Kphi/1 -> Sum2/2, Sum/2
  Kpsi/1 -> Sum2/3, Sum3/3, Sum1/3, Sum/3
  Ktheta/1 -> Sum1/2, Sum3/2

== system sim_UAV_Cascada/Sistema Quadrotor/DINÁMICA QUADROTOR/6 DoF ==
  Fuerzas : Inport
  Momentos : Inport  Port=2
  Cinematica : Subsystem
  Dinamica : Subsystem
  v_i : Outport
  r_i : Outport  Port=2
  Euler : Outport  Port=3
  Rib : Outport  Port=4
  Eulerdot : Outport  Port=5
  qib : Outport  Port=6
  v_b : Outport  Port=7
  wb_ib : Outport  Port=8
  a_b : Outport  Port=9
  wdot_b_ib : Outport  Port=10
  wires:
  Fuerzas/1 -> Dinamica/1(F_b)
  Momentos/1 -> Dinamica/2(M_b)
  Dinamica/1(v_b) -> v_b/1, Cinematica/1(v_b)
  Dinamica/2(wb_ib) -> wb_ib/1, Cinematica/2(wb_ib)
  Dinamica/3(wdot_b_ib) -> wdot_b_ib/1
  Dinamica/4(a_b) -> a_b/1
  Cinematica/1(Rib) -> Rib/1
  Cinematica/2(v_i) -> v_i/1
  Cinematica/3(r_i) -> r_i/1
  Cinematica/4(Euler) -> Euler/1
  Cinematica/5(Eulerdot) -> Eulerdot/1
  Cinematica/6(qib) -> qib/1

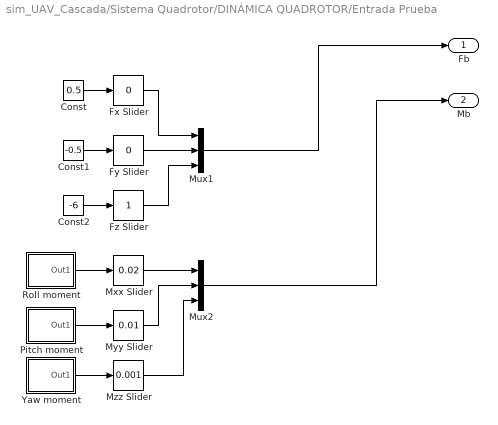
== system sim_UAV_Cascada/Sistema Quadrotor/DINÁMICA QUADROTOR/Entrada Prueba ==
  Const : Constant  Value=0.5
  Const1 : Constant  Value=-0.5
  Const2 : Constant  Value=-6
  Fx Slider : simulink/Math Operations/Slider Gain  low=-1  gain=0  high=1
  Fy Slider : simulink/Math Operations/Slider Gain  low=-1  gain=0  high=1
  Fz Slider : simulink/Math Operations/Slider Gain  low=-1  gain=1  high=1
  Mux1 : Mux  Inputs=3
  Mux2 : Mux  Inputs=3
  Mxx Slider : simulink/Math Operations/Slider Gain  low=-5  gain=0.02  high=10
  Myy Slider : simulink/Math Operations/Slider Gain  low=-10  gain=0.01  high=10
  Mzz Slider : simulink/Math Operations/Slider Gain  low=-1  gain=0.001  high=1
  Pitch moment : Subsystem  mask(timed input){t=[0 3 3 4 4 5 5  7.5 7.5 8.5 8.5 9.5 9.5 10], u=[0 0  1 1 -1 -1.005 0 0 -1 -1 1 1 0 0]*3.138/2}
      mask prompts: t "time values:"; u "input values"
      mask Display: plot(t,u)
  Roll moment : Subsystem  mask(timed input){t=[0 1 1 2 2  10], u=[1 1 -1 -.998  0 0]*3.144/2}
      mask prompts: t "time values:"; u "input values"
      mask Display: plot(t,u)
  Yaw moment : Subsystem  mask(timed input){t=[0 6 6 7 7 8 8 10], u=[0 0  -1 -1 1 1 0 0]*3.1/2}
      mask prompts: t "time values:"; u "input values"
      mask Display: plot(t,u)
  Fb : Outport
  Mb : Outport  Port=2
  wires:
  Fz Slider/1 -> Mux1/3
  Const/1 -> Fx Slider/1
  Myy Slider/1 -> Mux2/2
  Const1/1 -> Fy Slider/1
  Yaw moment/1(Out1) -> Mzz Slider/1
  Roll moment/1(Out1) -> Mxx Slider/1
  Mzz Slider/1 -> Mux2/3
  Fx Slider/1 -> Mux1/1
  Const2/1 -> Fz Slider/1
  Pitch moment/1(Out1) -> Myy Slider/1
  Fy Slider/1 -> Mux1/2
  Mxx Slider/1 -> Mux2/1
  Mux2/1 -> Mb/1
  Mux1/1 -> Fb/1

== system sim_UAV_Cascada/Sistema Quadrotor/DINÁMICA QUADROTOR/F ==
  Fm_b : Inport
  Fg_i : Constant  Value=[0;0;m*g]
  Fuerzas Suelo : MATLAB Function  TreatAsAtomicUnit=on
  Math Function : Math  Operator=transpose  SaturateOnIntegerOverflow=on
  Product : Product  Multiplication=Matrix(*)
  Product1 : Product  Multiplication=Matrix(*)
  Product2 : Product
  Fg_b : Outport
  Ks : Outport  Port=2
  wires:
  Fg_i/1 -> Fuerzas Suelo/1(Fg_i), Product/2
  [R] -> Math Function/1
  Math Function/1 -> Product/1
  Fuerzas Suelo/1(Ks) -> Product2/2, Ks/1
  Product1/1 -> Fuerzas Suelo/2(Fm_i)
  [R] -> Product1/1
  Fm_b/1 -> Product1/2
  Product/1 -> Product2/1
  Product2/1 -> Fg_b/1

== system sim_UAV_Cascada/Sistema Quadrotor/DINÁMICA QUADROTOR/6 DoF/Cinematica ==
  note: Cinemática del Cuadrirotor
  note: rdot_i = v_i
  note: Eulerdot = J wb_ib
  note: v_i = Rib v_b
  v_b : Inport
  wb_ib : Inport  Port=2
  "Calculo de matriz de coseno directores, angulos de Euler y cuaterniones" : Subsystem
  Integrator : Integrator  InitialCondition=r0_i
  Product2 : Product  Multiplication=Matrix(*)  RndMeth=Zero
  Rib : Outport
  v_i : Outport  Port=2
  r_i : Outport  Port=3
  Euler : Outport  Port=4
  Eulerdot : Outport  Port=5
  qib : Outport  Port=6
  wires:
  Product2/1 -> v_i/1, Integrator/1
  v_b/1 -> Product2/2
  Integrator/1 -> r_i/1
  "Calculo de matriz de coseno directores, angulos de Euler y cuaterniones"/2(Euler) -> Euler/1
  "Calculo de matriz de coseno directores, angulos de Euler y cuaterniones"/3(Eulerdot) -> Eulerdot/1
  "Calculo de matriz de coseno directores, angulos de Euler y cuaterniones"/4(qib) -> qib/1
  wb_ib/1 -> "Calculo de matriz de coseno directores, angulos de Euler y cuaterniones"/1(w_b)
  "Calculo de matriz de coseno directores, angulos de Euler y cuaterniones"/1(Rib) -> Rib/1, Product2/1

== system sim_UAV_Cascada/Sistema Quadrotor/DINÁMICA QUADROTOR/6 DoF/Dinamica ==
  note: Dinamica del Cuadridrotor
  note: vdot_b
  note: F_b = m( vdot_b + wb_ib x v_b)
  note: M_b = I wb_ib + wb_ib x (I wb_ib)
  F_b : Inport
  M_b : Inport  Port=2
  (wb_ib)x(v_b) : aerolibutil/3x3 Cross Product
  Calculo de wdot_b_ib : Subsystem
  Constant : Constant  Value=masa  OutDataTypeStr=Inherit: Inherit via back propagation
  Constant1 : Constant  Value=Inercia  OutDataTypeStr=Inherit: Inherit via back propagation
  Product3 : Product  Inputs=*/  SaturateOnIntegerOverflow=on  OutDataTypeStr=Inherit: Same as first input
  Sum : Sum  Inputs=-+|  SaturateOnIntegerOverflow=on
  integrator1 : Integrator  InitialCondition=v0_b
  integrator2 : Integrator  InitialCondition=w0b_ib
  v_b : Outport
  wb_ib : Outport  Port=2
  wdot_b_ib : Outport  Port=3
  a_b : Outport  Port=4
  wires:
  Calculo de wdot_b_ib/1(wdot_b_ib) -> integrator2/1, wdot_b_ib/1
  Constant/1 -> Product3/2
  Product3/1 -> Sum/2, a_b/1
  F_b/1 -> Product3/1
  M_b/1 -> Calculo de wdot_b_ib/3(Moments)
  Sum/1 -> integrator1/1
  integrator1/1 -> (wb_ib)x(v_b)/2, v_b/1
  integrator2/1 -> wb_ib/1, (wb_ib)x(v_b)/1, Calculo de wdot_b_ib/1(wb_ib)
  Constant1/1 -> Calculo de wdot_b_ib/2(I)
  (wb_ib)x(v_b)/1 -> Sum/1

== system sim_UAV_Cascada/Sistema Quadrotor/DINÁMICA QUADROTOR/Entrada Prueba/Pitch moment ==
  From Workspace : FromWorkspace  VariableName=[t',u']  SampleTime=0
  Out1 : Outport
  wires:
  From Workspace/1 -> Out1/1

== system sim_UAV_Cascada/Sistema Quadrotor/DINÁMICA QUADROTOR/Entrada Prueba/Roll moment ==
  From Workspace : FromWorkspace  VariableName=[t',u']  SampleTime=0
  Out1 : Outport
  wires:
  From Workspace/1 -> Out1/1

== system sim_UAV_Cascada/Sistema Quadrotor/DINÁMICA QUADROTOR/Entrada Prueba/Yaw moment ==
  From Workspace : FromWorkspace  VariableName=[t',u']  SampleTime=0
  Out1 : Outport
  wires:
  From Workspace/1 -> Out1/1

== system sim_UAV_Cascada/Sistema Quadrotor/DINÁMICA QUADROTOR/6 DoF/Cinematica/Calculo de matriz de coseno directores, angulos de Euler y cuaterniones ==
  w_b : Inport
  Direction Cosine Matrix to Quaternions : aerolibtransform2/Direction Cosine Matrix  to Quaternions
  Math Function : Math  Operator=transpose  SaturateOnIntegerOverflow=on
  Rotation Angles to Direction Cosine Matrix : aerolibtransform2/Rotation Angles to Direction Cosine Matrix  rotationOrder=ZYX
  Selector : Selector  InputPortWidth=3  Indices=[3 2 1]
  Subsystem : Subsystem
  phi theta psi : Integrator  InitialCondition=eul_0
  Rib : Outport
  Euler : Outport  Port=2
  Eulerdot : Outport  Port=3
  qib : Outport  Port=4
  wires:
  Selector/1 -> Rotation Angles to Direction Cosine Matrix/1
  phi theta psi/1 -> Selector/1, Euler/1, Subsystem/2(phi theta psi)
  Subsystem/1(phidot thetadot psidot) -> phi theta psi/1, Eulerdot/1
  w_b/1 -> Subsystem/1(wx wy wz)
  Rotation Angles to Direction Cosine Matrix/1 -> Math Function/1
  Direction Cosine Matrix to Quaternions/1 -> qib/1
  Math Function/1 -> Rib/1, Direction Cosine Matrix to Quaternions/1

== system sim_UAV_Cascada/Sistema Quadrotor/DINÁMICA QUADROTOR/6 DoF/Dinamica/Calculo de wdot_b_ib ==
  wb_ib : Inport
  I : Inport  Port=2
  Moments : Inport  Port=3
  (wb_ib)x(I(wb_ib)) : aerolibutil/3x3 Cross Product
  Calculo I*wb_ib : Subsystem
  Product4 : Product  Inputs=/*  Multiplication=Matrix(*)  SaturateOnIntegerOverflow=on  OutDataTypeStr=Inherit: Same as first input
  Sum2 : Sum  Inputs=+-  SaturateOnIntegerOverflow=on
  wdot_b_ib : Outport
  wires:
  Moments/1 -> Sum2/1
  Product4/1 -> wdot_b_ib/1
  wb_ib/1 -> (wb_ib)x(I(wb_ib))/1, Calculo I*wb_ib/2(wb_ib)
  Calculo I*wb_ib/1(I * wb_ib) -> (wb_ib)x(I(wb_ib))/2
  (wb_ib)x(I(wb_ib))/1 -> Sum2/2
  Sum2/1 -> Product4/2
  I/1 -> Product4/1, Calculo I*wb_ib/1(Inercia)

== system sim_UAV_Cascada/Sistema Quadrotor/DINÁMICA QUADROTOR/6 DoF/Cinematica/Calculo de matriz de coseno directores, angulos de Euler y cuaterniones/Subsystem ==
  wx wy wz : Inport
  phi theta psi : Inport  Port=2
  Mux1 : Mux  Inputs=[3 3 3]
  Mux2 : Mux  Inputs=3
  phidot : Fcn  Expr=u[1]+(u[2]*u[4]+u[3]*u[7])*(u[5]/u[8])
  psidot : Fcn  Expr=(u[2]*u[4]+u[3]*u[7])/u[8]
  sincos : Trigonometry  Operator=sincos
  thetadot : Fcn  Expr=u[2]*u[7]-u[3]*u[4]
  phidot thetadot psidot : Outport  InitialOutput=0
  wires:
  Mux1/1 -> psidot/1, phidot/1, thetadot/1
  wx wy wz/1 -> Mux1/1
  phi theta psi/1 -> sincos/1
  psidot/1 -> Mux2/3
  thetadot/1 -> Mux2/2
  phidot/1 -> Mux2/1
  Mux2/1 -> phidot thetadot psidot/1
  sincos/1 -> Mux1/2
  sincos/2 -> Mux1/3

== system sim_UAV_Cascada/Sistema Quadrotor/DINÁMICA QUADROTOR/6 DoF/Dinamica/Calculo de wdot_b_ib/Calculo I*wb_ib ==
  Inercia : Inport
  wb_ib : Inport  Port=2
  Product : Product  Multiplication=Matrix(*)  SaturateOnIntegerOverflow=on  InputSameDT=on  OutDataTypeStr=Inherit: Same as first input
  I * wb_ib : Outport
  wires:
  wb_ib/1 -> Product/2
  Inercia/1 -> Product/1
  Product/1 -> I * wb_ib/1

== matlab function sim_UAV_Cascada/Sistema Quadrotor/DINÁMICA QUADROTOR/F/Fuerzas Suelo ==
  data: Fg_i input; Fm_i input; Ks output
function Ks  = fcn(Fg_i,Fm_i)
%#codegen

if abs(Fm_i(3))<= abs(Fg_i(3))
    Ks = 0;
else
    Ks = 1;
end
